simulink model "closedloop_P"  (R2020b)
settings: Solver=ode45  StartTime=0.0  StopTime=10.0  RelTol=1e-3
undefined symbols (not defined in the file): B_e, J_e, K_a, K_e, K_p, K_t, mu_k, sat, T
settings Model: Creator=jasper  LastModifiedBy=jasper

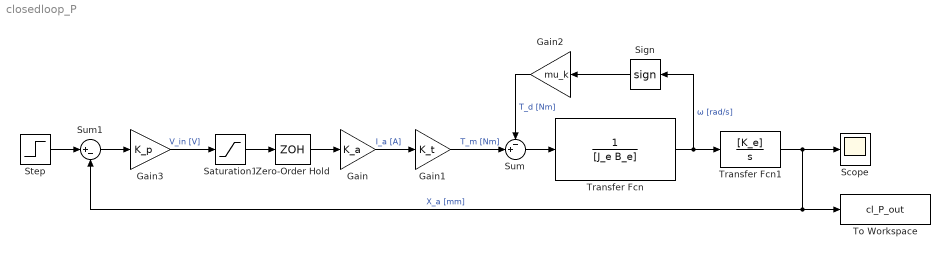
== system closedloop_P ==
  Gain : Gain  Gain=K_a
  Gain1 : Gain  Gain=K_t
  Gain2 : Gain  Gain=mu_k
  Gain3 : Gain  Gain=K_p
  Saturation1 : Saturate  UpperLimit=sat  LowerLimit=-sat  ZeroCross=off
  Scope : Scope
  Sign : Signum  ZeroCross=off
  Step : Step  SampleTime=0
  Sum : Sum  Inputs=-+|
  Sum1 : Sum  Inputs=|+-
  To Workspace : ToWorkspace  VariableName=cl_P_out  SaveFormat=Timeseries  SampleTime=-1
  Transfer Fcn : TransferFcn  Denominator=[J_e B_e]
  Transfer Fcn1 : TransferFcn  Numerator=[K_e]  Denominator=[1 0]
  Zero-Order Hold : ZeroOrderHold  SampleTime=T
  wires:
  Saturation1/1 -> Zero-Order Hold/1
  Zero-Order Hold/1 -> Gain/1
  Gain/1 -> Gain1/1  "I_a [A]"
  Gain1/1 -> Sum/2  "T_m [Nm]"
  Sum/1 -> Transfer Fcn/1
  Sign/1 -> Gain2/1
  Gain2/1 -> Sum/1  "T_d [Nm]"
  Transfer Fcn/1 -> Transfer Fcn1/1, Sign/1  "ω [rad/s]"
  Gain3/1 -> Saturation1/1  "V_in [V]"
  Sum1/1 -> Gain3/1
  Step/1 -> Sum1/1
  Transfer Fcn1/1 -> Scope/1, To Workspace/1, Sum1/2  "X_a [mm]"
